simulink model "eighth"  (R2021b)
settings: Solver=ode23s  StartTime=0.0  StopTime=2  RelTol=1e-3
libraries: spsBreakerLib x4, spsGroundLib x3, spsSeriesRLCBranchLib x3, spsDCVoltageSourceLib x2, spsDCMachineLib x1, spsVoltageMeasurementLib x1, spspowerguiLib x1
settings Model: Creator=minna  LastModifiedBy=minna
settings SolverCC: ZeroCrossAlgorithm=Adaptive
settings DebuggingCC: IgnoredZcDiagnostic=none

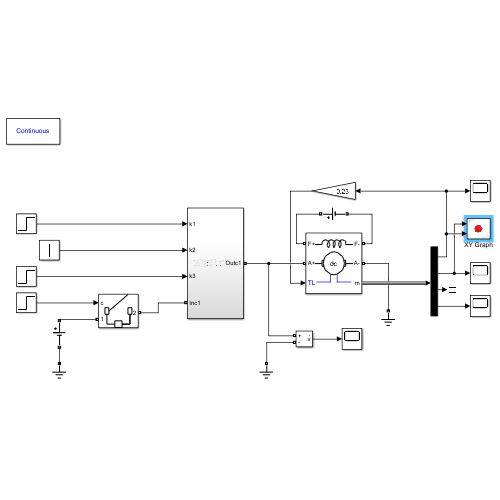
[thumbnail: Simulink's stored preview of the top-level diagram]
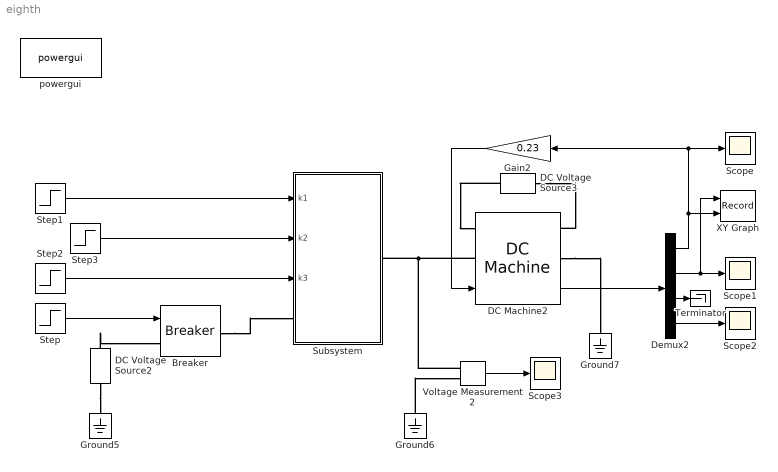
== system eighth ==
  Breaker : spsBreakerLib/Breaker  InitialState=0  SwitchingTimes="[1/60  5/60]"  External=on  BreakerResistance=0.1  SnubberResistance=1e6  SnubberCapacitance=inf  Measurements=None  MoreParameters=on  NoBreakLoop=off
      settings: SourceProductBaseCode=PS
  DC Machine2 : spsDCMachineLib/DC Machine  PresetModel=No  MechanicalLoad=Torque TL  FieldType=Wound  ShowDetailedParameters=on  MeasurementBus=off  RLa="[ 0.6717  0.001882]"  RLf="[ 30.72  3.166]"  Laf=0.2641  MachineConstant=Torque constant (N.m/A)  Ke=1.8  Kt=1.8  J=1.019  Bm=0  Tf=26.46  w0=1  Ifinit=7.64973958333333  TsPowergui=0  TsBlock=-1
  DC Voltage Source2 : spsDCVoltageSourceLib/DC Voltage Source  Amplitude=470  Measurements=None
  DC Voltage Source3 : spsDCVoltageSourceLib/DC Voltage Source  Amplitude=235  Measurements=None
  Demux2 : Demux
  Gain2 : Gain  Gain=0.23
  Ground5 : spsGroundLib/Ground  LConnTagsString=a
  Ground6 : spsGroundLib/Ground  LConnTagsString=a
  Ground7 : spsGroundLib/Ground  LConnTagsString=a
  Scope{,1..3} (4 alike) : Scope
  Step : Step  Time=0.2  SampleTime=0
  Step1 : Step  Time=0.481  SampleTime=0
  Step2 : Step  Time=0.827  SampleTime=0
  Step3 : Step  Time=0.680  SampleTime=0
  Subsystem : Subsystem
  Terminator : Terminator
  Voltage Measurement2 : spsVoltageMeasurementLib/Voltage Measurement  PhasorSimulation=off  OutputType=Complex  PSBequivalent=0
  XY Graph : Record  FileSettingsInternal="{\"entries\":[{\"content\":{\"excelSettings\":{\"content\":{},\"type\":\"Streamout.ExcelSettings\"}},\"type\":\"Streamout.FileSettingStorage\",\"uuid\":\"a846ec9c-767b-401b-a125-f1961f4e8617\"}],\"packageUris\":[\"http://schema.mathworks.com/mf0/streamout_blocks/R2020a\"],\"version\":\"1.0\"}"  Layout=[1 1]  SignalsInternal="{\"entries\":[{\"content\":{\"signals\":[{\"content\":{\"blockPath\":[\"eighth/XY Graph\"],\"channel\":[],\"dimensions\":[1],\"domain\":\"eighth/XY Graph\",\"lineColor\":\"#0072bd\",\"plots\":[],\"port\":1,\"sid\":[\"\"],\"signalID\":9376,\"signalName\":\"Demux2:2\"},\"type\":\"RecordBlkView.Signal\",\"uuid\":\"aafd61d2-d6d9-4e6c-a7a6-623e9779df97\"},{\"content\":{\"blockPath\":[\"eighth/XY Graph\"],\"channel\":[],\"dimensions\":[1],\"domain\":\"eighth/XY Graph\",\"lineColor\":\"#d95319\",\"plots\":[],\"port\":2,\"sid\":[\"\"],\"signalID\":9380,\"signalName\":\"Demux2:1\"},\"type\":\"RecordBlkView.Signal\",\"uuid\":\"7f1710d2-bfaa-468a-ba79-94a90518e088\"}]},\"type\":\"RecordBlkView.InputSignals\",\"uuid\":\"09f58f29-16ad-4b94-924b-db11702cc272\"}],\"packageUris\":[\"http://schema.mathworks.com/mf0/streamout_blocks/R2020a\"],\"version\":\"1.0\"}"  VisualizationBindings="{\"xyplotplugin\":{\"info\":[{\"series\":[],\"subplotID\":1}]}}"  CompatibilityTag=XY
  powergui : spspowerguiLib/powergui  Priority=1  SimulationMode=Continuous  SampleTime=50e-6  frequency=60  Iterations=50  frequencyindice=0  Pbase=100e6  ErrMax=1e-4  UnitsV=kV  UnitsW=MW  buscounter=0  FunctionMessages=off  echomessages=off  EnableUseOfTLC=off  CurrentSourceSwitches=off  DisableSnubberDevices=off  DisableRonSwitches=off  DisableVfSwitches=off  DisplayEquations=off  AutomaticDiscreteSolvers=off  SolverType=Tustin/Backward Euler (TBE)  Interpol=off  ExternalGateDelay=off  methode=off  Ts=100  x0status=blocks  SPID=on  SwTol=0  HookPort=off  NonlinearTolerance=1e-4  nMaxIteration=100  ContinueOnMaxIteration=off  RestoreLinks=warning  ResistiveCurrentMeasurement=off  Frange=[0:2:500]  Ylog=off  Xlog=on  ShowGrid=off  save=off  variable=ZData  structure=0  ZoomFFT=off  StartTime=0.0  cycles=1  DisplayStyle=1  fundamental=60  FreqAxis=off  MaxFrequency=1000  frequencyindicesteady=1  RmsSteady=1  display=off
  wires:
  Step/1 -> Breaker/1
  Step2/1 -> Subsystem/3(k3)
  Step3/1 -> Subsystem/2(k2)
  Step1/1 -> Subsystem/1(k1)
  Voltage Measurement2/1 -> Scope3/1
  DC Machine2/1 -> Demux2/1
  Demux2/4 -> Scope2/1
  Demux2/3 -> Terminator/1
  Demux2/2 -> XY Graph/1, Scope1/1
  Demux2/1 -> Gain2/1, Scope/1, XY Graph/2
  Gain2/1 -> DC Machine2/1
  connections:
  DC Voltage Source2/LConn1 -- Ground5/LConn1
  DC Voltage Source2/RConn1 -- Breaker/LConn1
  Breaker/RConn1 -- Subsystem/LConn1
  DC Machine2/LConn1 -- Subsystem/RConn1 -- Voltage Measurement2/LConn1
  Ground6/LConn1 -- Voltage Measurement2/LConn2
  DC Machine2/RConn1 -- Ground7/LConn1
  DC Voltage Source3/LConn1 -- DC Machine2/RConn2
  DC Voltage Source3/RConn1 -- DC Machine2/LConn2

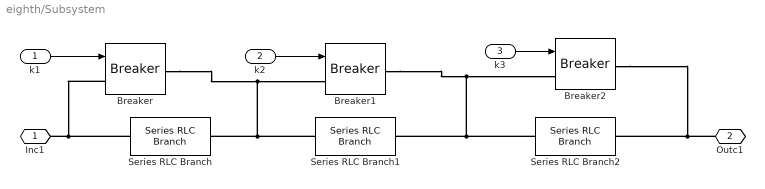
== system eighth/Subsystem ==
  k1 : Inport
  k2 : Inport  Port=2
  k3 : Inport  Port=3
  Breaker : spsBreakerLib/Breaker  InitialState=0  SwitchingTimes="[1/60  5/60]"  External=on  BreakerResistance=0.01  SnubberResistance=inf  SnubberCapacitance=inf  Measurements=None  MoreParameters=on  NoBreakLoop=off
      settings: SourceProductBaseCode=PS
  Breaker1 : spsBreakerLib/Breaker  InitialState=0  SwitchingTimes="[1/60  5/60]"  External=on  BreakerResistance=0.01  SnubberResistance=inf  SnubberCapacitance=inf  Measurements=None  MoreParameters=on  NoBreakLoop=off
      settings: SourceProductBaseCode=PS
  Breaker2 : spsBreakerLib/Breaker  InitialState=0  SwitchingTimes="[1/60  5/60]"  External=on  BreakerResistance=0.01  SnubberResistance=inf  SnubberCapacitance=inf  Measurements=None  MoreParameters=on  NoBreakLoop=off
      settings: SourceProductBaseCode=PS
  Series RLC Branch : spsSeriesRLCBranchLib/Series RLC Branch  LConnTagsString=__new0  RConnTagsString=__new0  BranchType=R  Resistance=0.813  Inductance=1e-3  SetiL0=off  InitialCurrent=0  Capacitance=1e-6  Setx0=off  InitialVoltage=0  Measurements=None
  Series RLC Branch1 : spsSeriesRLCBranchLib/Series RLC Branch  LConnTagsString=__new0  RConnTagsString=__new0  BranchType=R  Resistance=0.58  Inductance=1e-3  SetiL0=off  InitialCurrent=0  Capacitance=1e-6  Setx0=off  InitialVoltage=0  Measurements=None
  Series RLC Branch2 : spsSeriesRLCBranchLib/Series RLC Branch  LConnTagsString=__new0  RConnTagsString=__new0  BranchType=R  Resistance=0.41  Inductance=1e-3  SetiL0=off  InitialCurrent=0  Capacitance=1e-6  Setx0=off  InitialVoltage=0  Measurements=None
  Inc1 : PMIOPort  Side=Left
  Outc1 : PMIOPort  Port=2  Side=Right
  wires:
  k1/1 -> Breaker/1
  k2/1 -> Breaker1/1
  k3/1 -> Breaker2/1
  connections:
  Series RLC Branch/LConn1 -- Breaker/LConn1 -- Inc1/RConn1
  Outc1/RConn1 -- Breaker2/RConn1 -- Series RLC Branch2/RConn1
  Series RLC Branch1/LConn1 -- Breaker1/LConn1 -- Breaker/RConn1 -- Series RLC Branch/RConn1
  Series RLC Branch2/LConn1 -- Breaker2/LConn1 -- Breaker1/RConn1 -- Series RLC Branch1/RConn1
